simulink model "MotorSim_ReducedFidelityComparison"  (R2018a)
settings: Solver=VariableStepAuto  StartTime=0.0  StopTime=0.5  MaxStep=1/(PWM_Resolution*PWM_Frequency)  RelTol=1e-3
PreLoadFcn:
  | modelDir = fileparts(get_param(bdroot, 'FileName'));
  | addpath(fullfile(modelDir,'Parameters'));
  | addpath(fullfile(modelDir,'subsystems'));
  | 
  | Parameters_Model
  | Parameters_Simulation
InitFcn:
  | Parameters_Model
  | Parameters_Simulation
undefined symbols (not defined in the file or in its folder): EnableNoise, PWM_Duty, PWM_Frequency, PWM_Resolution, sensor_sigma2_current_sense
libraries: simulink x11
settings Model: Creator=Thomas  LastModifiedBy=Thomas

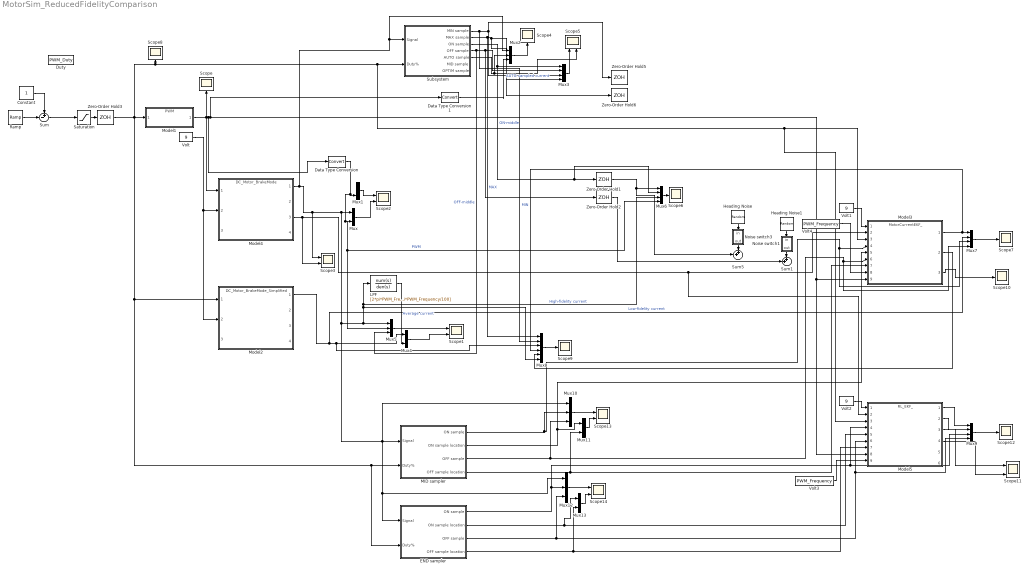
== system MotorSim_ReducedFidelityComparison ==
  Constant : Constant
  Data Type Conversion : DataTypeConversion  RndMeth=Round
  Data Type Conversion1 : DataTypeConversion  RndMeth=Round
  Duty : Constant  Value=PWM_Duty
  END sampler : Subsystem
  Heading Noise : RandomNumber  Variance=(0.02/3)^2  Seed=19  SampleTime=1/PWM_Frequency
  Heading Noise1 : RandomNumber  Variance=(0.02/3)^2  Seed=55  SampleTime=1/PWM_Frequency
  LPF : TransferFcn  Numerator=[2*pi*PWM_Frequency/100]  Denominator=[1 2*pi*PWM_Frequency/100]
  MID sampler : Subsystem
  Model1 : ModelReference  ModelNameDialog=PWM  SimulationMode=Normal  ModelReferenceVersion=1.19
  Model2 : ModelReference  ModelNameDialog=DC_Motor_BrakeMode_Simplified  SimulationMode=Normal  ModelReferenceVersion=1.19
  Model3 : ModelReference  ModelNameDialog=MotorCurrentEKF_  SimulationMode=Normal  ModelReferenceVersion=1.42
  Model4 : ModelReference  ModelNameDialog=DC_Motor_BrakeMode  SimulationMode=Normal  ModelReferenceVersion=1.16
  Model5 : ModelReference  ModelNameDialog=RL_EKF_  SimulationMode=Normal  ModelReferenceVersion=1.67
  Mux{,1,4,11,13} (5 alike) : Mux  Inputs=2
  Mux{2,5,10,12} (4 alike) : Mux  Inputs=3
  Mux{3,6..7,9} (4 alike) : Mux
  Mux8 : Mux  Inputs=6
  Noise switch1 : Subsystem
  Noise switch3 : Subsystem
  Ramp : simulink/Sources/Ramp  slope=10*0.8  start=0  InitialOutput=0.1
  Saturation : Saturate  UpperLimit=0.8  LowerLimit=0
  Scope{,4,6..10,12} (8 alike) : Scope
  Scope{1..3,5,11,13..14} (7 alike) : Scope  NumInputPorts=2
  Subsystem : Subsystem
  Sum : Sum  Inputs=+-|
  Sum1 : Sum  Inputs=++|
  Sum5 : Sum  Inputs=++|
  Volt : Constant  Value=9
  Volt1 : Constant  Value=9
  Volt2 : Constant  Value=9
  Volt3 : Constant  Value=PWM_Frequency
  Volt4 : Constant  Value=PWM_Frequency
  Zero-Order Hold{1..2,5..6} (4 alike) : ZeroOrderHold  SampleTime=1/PWM_Frequency
  Zero-Order Hold3 : ZeroOrderHold  SampleTime=500/PWM_Frequency
  wires:
  Volt/1 -> Model2/2, Model4/2
  Model4/1 -> Mux2/1, Subsystem/1(Signal), Scope3/1, Mux8/6, Mux6/3, LPF/1, Mux5/1, Mux12/1, END sampler/1(Signal), Mux10/1, MID sampler/1(Signal), Mux/1  "High-fidelity current"
  Mux/1 -> Scope2/2
  Mux1/1 -> Scope2/1
  Model1/1 -> Model3/9, Model5/8, Data Type Conversion1/1, Data Type Conversion/1, Scope/1, Model4/1
  Data Type Conversion/1 -> Mux6/4, Mux5/2, Mux/2, Mux1/2  "PWM"
  Mux2/1 -> Scope4/1
  Data Type Conversion1/1 -> Mux2/3
  Mux3/1 -> Scope5/1
  Subsystem/4(OFF sample) -> Mux5/3, Zero-Order Hold2/1, Mux3/2  "OFF-middle"
  Subsystem/5(AUTO sample) -> Mux2/2, Scope5/2  "AUTO sampled current"
  Subsystem/1(MIN sample) -> Mux8/2, Zero-Order Hold5/1, Mux3/3  "MIN"
  Subsystem/2(MAX sample) -> Mux8/1, Zero-Order Hold6/1, Mux3/4  "MAX"
  Subsystem/3(ON sample) -> Mux6/2, Zero-Order Hold1/1, Mux3/1  "ON-middle"
  Model2/1 -> Mux7/2, Mux8/3, Mux4/1  "Low-fidelity current"
  Mux5/1 -> Scope1/1
  Mux4/1 -> Scope1/2
  LPF/1 -> Mux4/2  "Average current"
  Mux6/1 -> Scope6/1
  Zero-Order Hold1/1 -> Sum5/2, Mux6/1
  Zero-Order Hold2/1 -> Sum1/2
  Volt1/1 -> Model3/1
  Model3/1 -> Mux8/4, Mux7/1
  Mux7/1 -> Scope7/1
  Heading Noise/1 -> Noise switch3/1(in)
  Noise switch3/1(out) -> Sum5/1
  Heading Noise1/1 -> Noise switch1/1(in)
  Noise switch1/1(out) -> Sum1/1
  Mux8/1 -> Scope9/1
  Saturation/1 -> Zero-Order Hold3/1
  Model3/3 -> Scope10/1
  Zero-Order Hold3/1 -> END sampler/2(Duty%), MID sampler/2(Duty%), Model2/1, Scope8/1, Model3/3, Model5/3, Subsystem/2(Duty%), Model1/1
  Model3/2 -> Mux8/5
  Volt2/1 -> Model5/1
  Model5/1 -> Mux9/1
  Model5/3 -> Scope11/1
  Mux9/1 -> Scope12/1
  MID sampler/3(OFF sample) -> Mux7/4, Model3/6, Mux10/3
  MID sampler/1(ON sample) -> Mux7/3, Model3/4, Mux10/2
  Model5/4 -> Scope11/2
  MID sampler/2(ON sample location) -> Model3/5, Mux11/1
  Mux10/1 -> Scope13/1
  Mux11/1 -> Scope13/2
  MID sampler/4(OFF sample location) -> Mux11/2, Model3/7
  Model4/3 -> Model3/2, Model5/2, Scope3/2
  Ramp/1 -> Sum/2
  Sum/1 -> Saturation/1
  Constant/1 -> Sum/1
  Model5/2 -> Mux9/2
  END sampler/1(ON sample) -> Model5/4, Mux9/3, Mux12/2
  END sampler/2(ON sample location) -> Mux13/1, Model5/5
  END sampler/3(OFF sample) -> Mux9/4, Model5/6, Mux12/3
  END sampler/4(OFF sample location) -> Mux13/2, Model5/7
  Mux13/1 -> Scope14/2
  Mux12/1 -> Scope14/1
  Volt3/1 -> Model5/9
  Volt4/1 -> Model3/8

== system MotorSim_ReducedFidelityComparison/END sampler ==
  Signal : Inport
  Duty% : Inport  Port=2  OutDataTypeStr=double
  OFF-end sampler : Subsystem
  ON-end sampler : Subsystem
  ON sample : Outport
  ON sample location : Outport  Port=2
  OFF sample : Outport  Port=3
  OFF sample location : Outport  Port=4
  wires:
  Signal/1 -> OFF-end sampler/1(Signal), ON-end sampler/1(Signal)
  ON-end sampler/1(Sample) -> ON sample/1
  Duty%/1 -> ON-end sampler/2(Duty%)
  OFF-end sampler/1(Sample) -> OFF sample/1
  ON-end sampler/2(Sample location) -> ON sample location/1
  OFF-end sampler/2(Sample location) -> OFF sample location/1

== system MotorSim_ReducedFidelityComparison/MID sampler ==
  Signal : Inport
  Duty% : Inport  Port=2  OutDataTypeStr=double
  OFF-mid sampler : Subsystem
  ON-mid sampler : Subsystem
  ON sample : Outport
  ON sample location : Outport  Port=2
  OFF sample : Outport  Port=3
  OFF sample location : Outport  Port=4
  wires:
  Signal/1 -> OFF-mid sampler/1(Signal), ON-mid sampler/1(Signal)
  ON-mid sampler/1(Sample) -> ON sample/1
  Duty%/1 -> OFF-mid sampler/2(Duty%), ON-mid sampler/2(Duty%)
  OFF-mid sampler/1(Sample) -> OFF sample/1
  ON-mid sampler/2(Sample location) -> ON sample location/1
  OFF-mid sampler/2(Sample location) -> OFF sample location/1

== system MotorSim_ReducedFidelityComparison/Noise switch1 ==
  in : Inport
  Enable noise : Constant  Value=EnableNoise
  No noise : Constant  Value=0
  Switch : Switch  Criteria=u2 > Threshold
  out : Outport
  wires:
  No noise/1 -> Switch/3
  Switch/1 -> out/1
  Enable noise/1 -> Switch/2
  in/1 -> Switch/1

== system MotorSim_ReducedFidelityComparison/Noise switch3 ==
  in : Inport
  Enable noise : Constant  Value=EnableNoise
  No noise : Constant  Value=0
  Switch : Switch  Criteria=u2 > Threshold
  out : Outport
  wires:
  No noise/1 -> Switch/3
  Switch/1 -> out/1
  Enable noise/1 -> Switch/2
  in/1 -> Switch/1

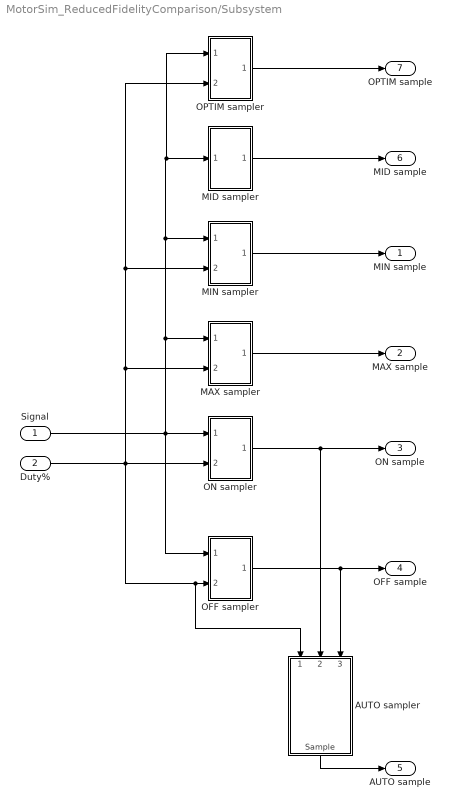
== system MotorSim_ReducedFidelityComparison/Subsystem ==
  Signal : Inport
  Duty% : Inport  Port=2  OutDataTypeStr=double
  AUTO sampler : Subsystem
  MAX sampler : Subsystem
  MID sampler : Subsystem
  MIN sampler : Subsystem
  OFF sampler : Subsystem
  ON sampler : Subsystem
  OPTIM sampler : Subsystem
  MIN sample : Outport
  MAX sample : Outport  Port=2
  ON sample : Outport  Port=3
  OFF sample : Outport  Port=4
  AUTO sample : Outport  Port=5
  MID sample : Outport  Port=6
  OPTIM sample : Outport  Port=7
  wires:
  Signal/1 -> MAX sampler/1(Signal), MIN sampler/1(Signal), OPTIM sampler/1(Signal), MID sampler/1(Signal), OFF sampler/1(Signal), ON sampler/1(Signal)
  ON sampler/1(Sample) -> AUTO sampler/2(ON sample), ON sample/1
  OFF sampler/1(Sample) -> AUTO sampler/3(OFF sample), OFF sample/1
  AUTO sampler/1(Sample) -> AUTO sample/1
  Duty%/1 -> MIN sampler/2(Duty%), OPTIM sampler/2(Duty%), MAX sampler/2(Duty%), AUTO sampler/1(Duty%), OFF sampler/2(Duty%), ON sampler/2(Duty%)
  MAX sampler/1(Sample) -> MAX sample/1
  MIN sampler/1(Sample) -> MIN sample/1
  MID sampler/1(Sample) -> MID sample/1
  OPTIM sampler/1(Sample) -> OPTIM sample/1

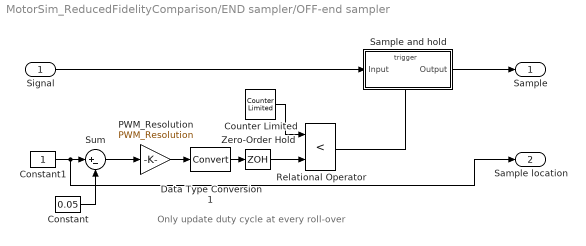
== system MotorSim_ReducedFidelityComparison/END sampler/OFF-end sampler ==
  note: Only update duty cycle at every roll-over
  Signal : Inport
  Constant : Constant  Value=0.05
  Constant1 : Constant
  Counter Limited : simulink/Sources/Counter Limited  uplimit=PWM_Resolution-1  tsamp=1/(PWM_Resolution*PWM_Frequency)
  Data Type Conversion1 : DataTypeConversion  RndMeth=Round
  PWM_Resolution : Gain  Gain=PWM_Resolution
  Relational Operator : RelationalOperator  Operator=<  OutDataTypeStr=boolean  RndMeth=Simplest
  Sample and hold : Subsystem
  Sum : Sum  Inputs=|+-
  Zero-Order Hold : ZeroOrderHold  SampleTime=1/PWM_Frequency
  Sample : Outport
  Sample location : Outport  Port=2
  wires:
  Relational Operator/1 -> Sample and hold/Trigger
  Zero-Order Hold/1 -> Relational Operator/2
  Counter Limited/1 -> Relational Operator/1
  Signal/1 -> Sample and hold/1(Input)
  Data Type Conversion1/1 -> Zero-Order Hold/1
  Sum/1 -> PWM_Resolution/1
  Sample and hold/1(Output) -> Sample/1
  Constant/1 -> Sum/2
  Constant1/1 -> Sample location/1, Sum/1
  PWM_Resolution/1 -> Data Type Conversion1/1

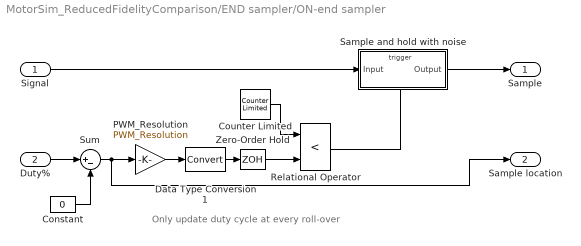
== system MotorSim_ReducedFidelityComparison/END sampler/ON-end sampler ==
  note: Only update duty cycle at every roll-over
  Signal : Inport
  Duty% : Inport  Port=2  OutDataTypeStr=double
  Constant : Constant  Value=0
  Counter Limited : simulink/Sources/Counter Limited  uplimit=PWM_Resolution-1  tsamp=1/(PWM_Resolution*PWM_Frequency)
  Data Type Conversion1 : DataTypeConversion  RndMeth=Round
  PWM_Resolution : Gain  Gain=PWM_Resolution
  Relational Operator : RelationalOperator  Operator=<  OutDataTypeStr=boolean  RndMeth=Simplest
  Sample and hold with noise : Subsystem
  Sum : Sum  Inputs=|+-
  Zero-Order Hold : ZeroOrderHold  SampleTime=1/PWM_Frequency
  Sample : Outport
  Sample location : Outport  Port=2
  wires:
  Relational Operator/1 -> Sample and hold with noise/Trigger
  Zero-Order Hold/1 -> Relational Operator/2
  Counter Limited/1 -> Relational Operator/1
  Signal/1 -> Sample and hold with noise/1(Input)
  Data Type Conversion1/1 -> Zero-Order Hold/1
  Sum/1 -> PWM_Resolution/1, Sample location/1
  Sample and hold with noise/1(Output) -> Sample/1
  Constant/1 -> Sum/2
  Duty%/1 -> Sum/1
  PWM_Resolution/1 -> Data Type Conversion1/1

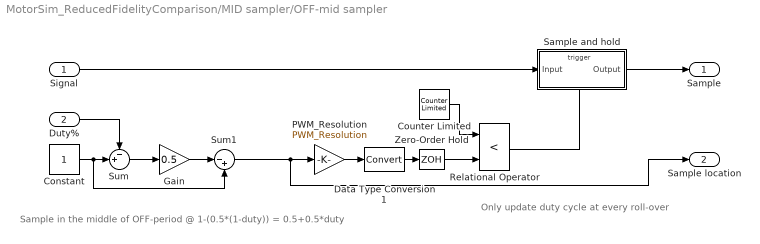
== system MotorSim_ReducedFidelityComparison/MID sampler/OFF-mid sampler ==
  note: Only update duty cycle at every roll-over
  note: Sample in the middle of OFF-period @ 1-(0.5*(1-duty)) = 0.5+0.5*duty
  Signal : Inport
  Duty% : Inport  Port=2  OutDataTypeStr=double
  Constant : Constant
  Counter Limited : simulink/Sources/Counter Limited  uplimit=PWM_Resolution-1  tsamp=1/(PWM_Resolution*PWM_Frequency)
  Data Type Conversion1 : DataTypeConversion  RndMeth=Round
  Gain : Gain  Gain=0.5
  PWM_Resolution : Gain  Gain=PWM_Resolution
  Relational Operator : RelationalOperator  Operator=<  OutDataTypeStr=boolean  RndMeth=Simplest
  Sample and hold : Subsystem
  Sum : Sum  Inputs=-+|
  Sum1 : Sum  Inputs=|-+
  Zero-Order Hold : ZeroOrderHold  SampleTime=1/PWM_Frequency
  Sample : Outport
  Sample location : Outport  Port=2
  wires:
  Relational Operator/1 -> Sample and hold/Trigger
  Zero-Order Hold/1 -> Relational Operator/2
  Counter Limited/1 -> Relational Operator/1
  Signal/1 -> Sample and hold/1(Input)
  Data Type Conversion1/1 -> Zero-Order Hold/1
  Sum1/1 -> PWM_Resolution/1, Sample location/1
  Sample and hold/1(Output) -> Sample/1
  PWM_Resolution/1 -> Data Type Conversion1/1
  Duty%/1 -> Sum/1
  Sum/1 -> Gain/1
  Constant/1 -> Sum1/2, Sum/2
  Gain/1 -> Sum1/1

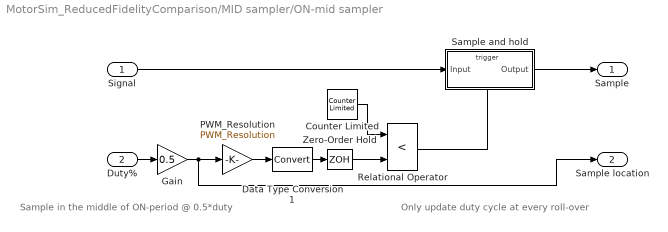
== system MotorSim_ReducedFidelityComparison/MID sampler/ON-mid sampler ==
  note: Sample in the middle of ON-period @ 0.5*duty
  note: Only update duty cycle at every roll-over
  Signal : Inport
  Duty% : Inport  Port=2  OutDataTypeStr=double
  Counter Limited : simulink/Sources/Counter Limited  uplimit=PWM_Resolution-1  tsamp=1/(PWM_Resolution*PWM_Frequency)
  Data Type Conversion1 : DataTypeConversion  RndMeth=Round
  Gain : Gain  Gain=0.5
  PWM_Resolution : Gain  Gain=PWM_Resolution
  Relational Operator : RelationalOperator  Operator=<  OutDataTypeStr=boolean  RndMeth=Simplest
  Sample and hold : Subsystem
  Zero-Order Hold : ZeroOrderHold  SampleTime=1/PWM_Frequency
  Sample : Outport
  Sample location : Outport  Port=2
  wires:
  Relational Operator/1 -> Sample and hold/Trigger
  Zero-Order Hold/1 -> Relational Operator/2
  Counter Limited/1 -> Relational Operator/1
  Signal/1 -> Sample and hold/1(Input)
  Data Type Conversion1/1 -> Zero-Order Hold/1
  Gain/1 -> PWM_Resolution/1, Sample location/1
  Sample and hold/1(Output) -> Sample/1
  Duty%/1 -> Gain/1
  PWM_Resolution/1 -> Data Type Conversion1/1

== system MotorSim_ReducedFidelityComparison/Subsystem/AUTO sampler ==
  Duty% : Inport  OutDataTypeStr=double
  ON sample : Inport  Port=2
  OFF sample : Inport  Port=3
  Switch : Switch  Threshold=0.5
  Sample : Outport
  wires:
  Duty%/1 -> Switch/2
  ON sample/1 -> Switch/1
  OFF sample/1 -> Switch/3
  Switch/1 -> Sample/1

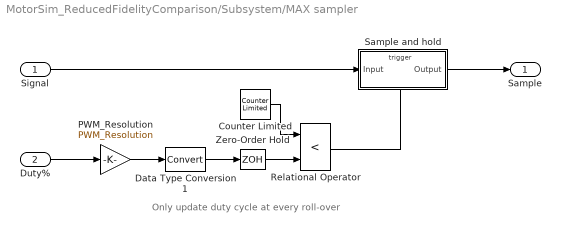
== system MotorSim_ReducedFidelityComparison/Subsystem/MAX sampler ==
  note: Only update duty cycle at every roll-over
  Signal : Inport
  Duty% : Inport  Port=2  OutDataTypeStr=double
  Counter Limited : simulink/Sources/Counter Limited  uplimit=PWM_Resolution-1  tsamp=1/(PWM_Resolution*PWM_Frequency)
  Data Type Conversion1 : DataTypeConversion  RndMeth=Round
  PWM_Resolution : Gain  Gain=PWM_Resolution
  Relational Operator : RelationalOperator  Operator=<  OutDataTypeStr=boolean  RndMeth=Simplest
  Sample and hold : Subsystem
  Zero-Order Hold : ZeroOrderHold  SampleTime=1/PWM_Frequency
  Sample : Outport
  wires:
  Relational Operator/1 -> Sample and hold/Trigger
  Zero-Order Hold/1 -> Relational Operator/2
  Counter Limited/1 -> Relational Operator/1
  Signal/1 -> Sample and hold/1(Input)
  Data Type Conversion1/1 -> Zero-Order Hold/1
  PWM_Resolution/1 -> Data Type Conversion1/1
  Sample and hold/1(Output) -> Sample/1
  Duty%/1 -> PWM_Resolution/1

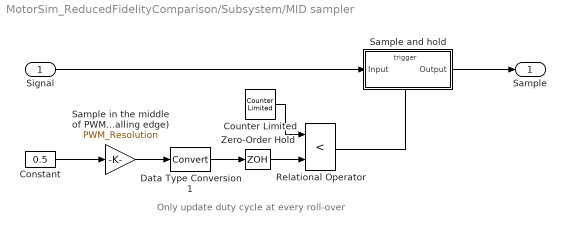
== system MotorSim_ReducedFidelityComparison/Subsystem/MID sampler ==
  note: Only update duty cycle at every roll-over
  Signal : Inport
  Constant : Constant  Value=0.5
  Counter Limited : simulink/Sources/Counter Limited  uplimit=PWM_Resolution-1  tsamp=1/(PWM_Resolution*PWM_Frequency)
  Data Type Conversion1 : DataTypeConversion  RndMeth=Round
  Relational Operator : RelationalOperator  Operator=<  OutDataTypeStr=boolean  RndMeth=Simplest
  Sample and hold : Subsystem
  Sample in the middle of PWM cycle (50% duty cycle falling edge) : Gain  Gain=PWM_Resolution
  Zero-Order Hold : ZeroOrderHold  SampleTime=1/PWM_Frequency
  Sample : Outport
  wires:
  Relational Operator/1 -> Sample and hold/Trigger
  Zero-Order Hold/1 -> Relational Operator/2
  Counter Limited/1 -> Relational Operator/1
  Signal/1 -> Sample and hold/1(Input)
  Data Type Conversion1/1 -> Zero-Order Hold/1
  Sample in the middle of PWM cycle (50% duty cycle falling edge)/1 -> Data Type Conversion1/1
  Sample and hold/1(Output) -> Sample/1
  Constant/1 -> Sample in the middle of PWM cycle (50% duty cycle falling edge)/1

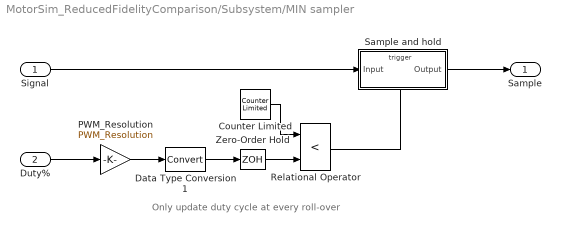
== system MotorSim_ReducedFidelityComparison/Subsystem/MIN sampler ==
  note: Only update duty cycle at every roll-over
  Signal : Inport
  Duty% : Inport  Port=2  OutDataTypeStr=double
  Counter Limited : simulink/Sources/Counter Limited  uplimit=PWM_Resolution-1  tsamp=1/(PWM_Resolution*PWM_Frequency)
  Data Type Conversion1 : DataTypeConversion  RndMeth=Round
  PWM_Resolution : Gain  Gain=PWM_Resolution
  Relational Operator : RelationalOperator  Operator=<  OutDataTypeStr=boolean  RndMeth=Simplest
  Sample and hold : Subsystem
  Zero-Order Hold : ZeroOrderHold  SampleTime=1/PWM_Frequency
  Sample : Outport
  wires:
  Relational Operator/1 -> Sample and hold/Trigger
  Zero-Order Hold/1 -> Relational Operator/2
  Counter Limited/1 -> Relational Operator/1
  Signal/1 -> Sample and hold/1(Input)
  Data Type Conversion1/1 -> Zero-Order Hold/1
  PWM_Resolution/1 -> Data Type Conversion1/1
  Sample and hold/1(Output) -> Sample/1
  Duty%/1 -> PWM_Resolution/1

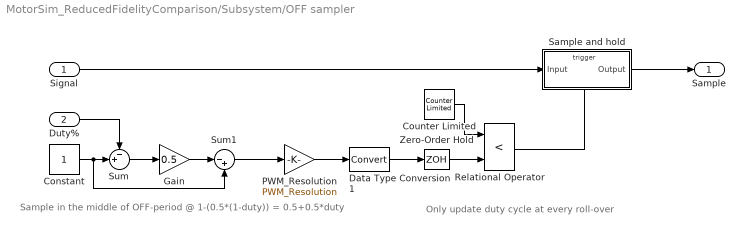
== system MotorSim_ReducedFidelityComparison/Subsystem/OFF sampler ==
  note: Sample in the middle of OFF-period @ 1-(0.5*(1-duty)) = 0.5+0.5*duty
  note: Only update duty cycle at every roll-over
  Signal : Inport
  Duty% : Inport  Port=2  OutDataTypeStr=double
  Constant : Constant
  Counter Limited : simulink/Sources/Counter Limited  uplimit=PWM_Resolution-1  tsamp=1/(PWM_Resolution*PWM_Frequency)
  Data Type Conversion1 : DataTypeConversion  RndMeth=Round
  Gain : Gain  Gain=0.5
  PWM_Resolution : Gain  Gain=PWM_Resolution
  Relational Operator : RelationalOperator  Operator=<  OutDataTypeStr=boolean  RndMeth=Simplest
  Sample and hold : Subsystem
  Sum : Sum  Inputs=-+|
  Sum1 : Sum  Inputs=|-+
  Zero-Order Hold : ZeroOrderHold  SampleTime=1/PWM_Frequency
  Sample : Outport
  wires:
  Relational Operator/1 -> Sample and hold/Trigger
  Zero-Order Hold/1 -> Relational Operator/2
  Counter Limited/1 -> Relational Operator/1
  Signal/1 -> Sample and hold/1(Input)
  Duty%/1 -> Sum/1
  Data Type Conversion1/1 -> Zero-Order Hold/1
  PWM_Resolution/1 -> Data Type Conversion1/1
  Sample and hold/1(Output) -> Sample/1
  Sum/1 -> Gain/1
  Constant/1 -> Sum1/2, Sum/2
  Gain/1 -> Sum1/1
  Sum1/1 -> PWM_Resolution/1

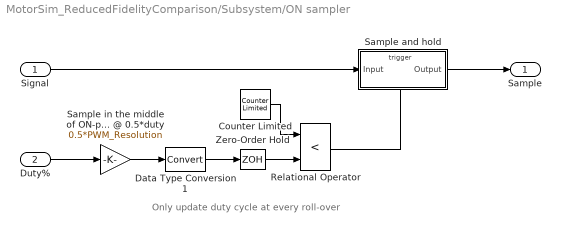
== system MotorSim_ReducedFidelityComparison/Subsystem/ON sampler ==
  note: Only update duty cycle at every roll-over
  Signal : Inport
  Duty% : Inport  Port=2  OutDataTypeStr=double
  Counter Limited : simulink/Sources/Counter Limited  uplimit=PWM_Resolution-1  tsamp=1/(PWM_Resolution*PWM_Frequency)
  Data Type Conversion1 : DataTypeConversion  RndMeth=Round
  Relational Operator : RelationalOperator  Operator=<  OutDataTypeStr=boolean  RndMeth=Simplest
  Sample and hold : Subsystem
  Sample in the middle of ON-period @ 0.5*duty : Gain  Gain=0.5*PWM_Resolution
  Zero-Order Hold : ZeroOrderHold  SampleTime=1/PWM_Frequency
  Sample : Outport
  wires:
  Relational Operator/1 -> Sample and hold/Trigger
  Zero-Order Hold/1 -> Relational Operator/2
  Counter Limited/1 -> Relational Operator/1
  Signal/1 -> Sample and hold/1(Input)
  Data Type Conversion1/1 -> Zero-Order Hold/1
  Sample in the middle of ON-period @ 0.5*duty/1 -> Data Type Conversion1/1
  Sample and hold/1(Output) -> Sample/1
  Duty%/1 -> Sample in the middle of ON-period @ 0.5*duty/1

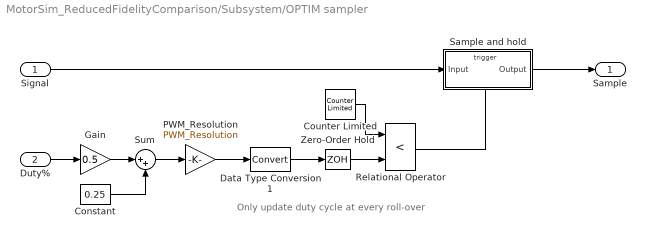
== system MotorSim_ReducedFidelityComparison/Subsystem/OPTIM sampler ==
  note: Only update duty cycle at every roll-over
  Signal : Inport
  Duty% : Inport  Port=2  OutDataTypeStr=double
  Constant : Constant  Value=0.25
  Counter Limited : simulink/Sources/Counter Limited  uplimit=PWM_Resolution-1  tsamp=1/(PWM_Resolution*PWM_Frequency)
  Data Type Conversion1 : DataTypeConversion  RndMeth=Round
  Gain : Gain  Gain=0.5
  PWM_Resolution : Gain  Gain=PWM_Resolution
  Relational Operator : RelationalOperator  Operator=<  OutDataTypeStr=boolean  RndMeth=Simplest
  Sample and hold : Subsystem
  Sum : Sum  Inputs=|++
  Zero-Order Hold : ZeroOrderHold  SampleTime=1/PWM_Frequency
  Sample : Outport
  wires:
  Relational Operator/1 -> Sample and hold/Trigger
  Zero-Order Hold/1 -> Relational Operator/2
  Counter Limited/1 -> Relational Operator/1
  Signal/1 -> Sample and hold/1(Input)
  Data Type Conversion1/1 -> Zero-Order Hold/1
  PWM_Resolution/1 -> Data Type Conversion1/1
  Sample and hold/1(Output) -> Sample/1
  Sum/1 -> PWM_Resolution/1
  Constant/1 -> Sum/2
  Duty%/1 -> Gain/1
  Gain/1 -> Sum/1

== system MotorSim_ReducedFidelityComparison/END sampler/OFF-end sampler/Sample and hold ==
  Input : Inport
  Trigger : TriggerPort  VariantControl=Variant  PortDimensions=1
  Noise : RandomNumber  Variance=sensor_sigma2_current_sense  Seed=35
  Noise switch : Subsystem
  Sum2 : Sum  Inputs=++|
  Output : Outport
  wires:
  Noise/1 -> Noise switch/1(in)
  Input/1 -> Sum2/2
  Noise switch/1(out) -> Sum2/1
  Sum2/1 -> Output/1

== system MotorSim_ReducedFidelityComparison/END sampler/ON-end sampler/Sample and hold with noise ==
  Input : Inport
  Trigger : TriggerPort  TriggerType=falling  VariantControl=Variant  PortDimensions=1
  Noise : RandomNumber  Variance=sensor_sigma2_current_sense  Seed=55
  Noise switch : Subsystem
  Sum2 : Sum  Inputs=++|
  Output : Outport
  wires:
  Noise/1 -> Noise switch/1(in)
  Input/1 -> Sum2/2
  Noise switch/1(out) -> Sum2/1
  Sum2/1 -> Output/1

== system MotorSim_ReducedFidelityComparison/MID sampler/OFF-mid sampler/Sample and hold ==
  Input : Inport
  Trigger : TriggerPort  TriggerType=falling  VariantControl=Variant  PortDimensions=1
  Noise : RandomNumber  Variance=sensor_sigma2_current_sense  Seed=35
  Noise switch : Subsystem
  Sum2 : Sum  Inputs=++|
  Output : Outport
  wires:
  Sum2/1 -> Output/1
  Input/1 -> Sum2/2
  Noise/1 -> Noise switch/1(in)
  Noise switch/1(out) -> Sum2/1

== system MotorSim_ReducedFidelityComparison/MID sampler/ON-mid sampler/Sample and hold ==
  Input : Inport
  Trigger : TriggerPort  TriggerType=falling  VariantControl=Variant  PortDimensions=1
  Noise : RandomNumber  Variance=sensor_sigma2_current_sense  Seed=55
  Noise switch : Subsystem
  Sum2 : Sum  Inputs=++|
  Output : Outport
  wires:
  Sum2/1 -> Output/1
  Input/1 -> Sum2/2
  Noise/1 -> Noise switch/1(in)
  Noise switch/1(out) -> Sum2/1

== system MotorSim_ReducedFidelityComparison/Subsystem/MAX sampler/Sample and hold ==
  Input : Inport
  Trigger : TriggerPort  TriggerType=falling  VariantControl=Variant  PortDimensions=1
  Output : Outport
  wires:
  Input/1 -> Output/1

== system MotorSim_ReducedFidelityComparison/Subsystem/MID sampler/Sample and hold ==
  Input : Inport
  Trigger : TriggerPort  TriggerType=falling  VariantControl=Variant  PortDimensions=1
  Output : Outport
  wires:
  Input/1 -> Output/1

== system MotorSim_ReducedFidelityComparison/Subsystem/MIN sampler/Sample and hold ==
  Input : Inport
  Trigger : TriggerPort  VariantControl=Variant  PortDimensions=1
  Output : Outport
  wires:
  Input/1 -> Output/1

== system MotorSim_ReducedFidelityComparison/Subsystem/OFF sampler/Sample and hold ==
  Input : Inport
  Trigger : TriggerPort  TriggerType=falling  VariantControl=Variant  PortDimensions=1
  Output : Outport
  wires:
  Input/1 -> Output/1

== system MotorSim_ReducedFidelityComparison/Subsystem/ON sampler/Sample and hold ==
  Input : Inport
  Trigger : TriggerPort  TriggerType=falling  VariantControl=Variant  PortDimensions=1
  Output : Outport
  wires:
  Input/1 -> Output/1

== system MotorSim_ReducedFidelityComparison/Subsystem/OPTIM sampler/Sample and hold ==
  Input : Inport
  Trigger : TriggerPort  TriggerType=falling  VariantControl=Variant  PortDimensions=1
  Output : Outport
  wires:
  Input/1 -> Output/1

== system MotorSim_ReducedFidelityComparison/END sampler/OFF-end sampler/Sample and hold/Noise switch ==
  in : Inport
  Enable noise : Constant  Value=EnableNoise
  No noise : Constant  Value=0
  Switch : Switch  Criteria=u2 > Threshold
  out : Outport
  wires:
  No noise/1 -> Switch/3
  Switch/1 -> out/1
  Enable noise/1 -> Switch/2
  in/1 -> Switch/1

== system MotorSim_ReducedFidelityComparison/END sampler/ON-end sampler/Sample and hold with noise/Noise switch ==
  in : Inport
  Enable noise : Constant  Value=EnableNoise
  No noise : Constant  Value=0
  Switch : Switch  Criteria=u2 > Threshold
  out : Outport
  wires:
  No noise/1 -> Switch/3
  Switch/1 -> out/1
  Enable noise/1 -> Switch/2
  in/1 -> Switch/1

== system MotorSim_ReducedFidelityComparison/MID sampler/OFF-mid sampler/Sample and hold/Noise switch ==
  in : Inport
  Enable noise : Constant  Value=EnableNoise
  No noise : Constant  Value=0
  Switch : Switch  Criteria=u2 > Threshold
  out : Outport
  wires:
  No noise/1 -> Switch/3
  Switch/1 -> out/1
  Enable noise/1 -> Switch/2
  in/1 -> Switch/1

== system MotorSim_ReducedFidelityComparison/MID sampler/ON-mid sampler/Sample and hold/Noise switch ==
  in : Inport
  Enable noise : Constant  Value=EnableNoise
  No noise : Constant  Value=0
  Switch : Switch  Criteria=u2 > Threshold
  out : Outport
  wires:
  No noise/1 -> Switch/3
  Switch/1 -> out/1
  Enable noise/1 -> Switch/2
  in/1 -> Switch/1
